simulink model "motor"  (R2017b)
settings: Solver=VariableStepAuto  StartTime=0.0  StopTime=10.0  RelTol=1e-3
values from neighbouring files (symbols this model uses):
  k1 = minium_chro(1)    [GA_fuzzy.m]    (also in GA_fuzzy_fitfun.m = chro(1))
  k2 = minium_chro(2)    [GA_fuzzy.m]    (also in GA_fuzzy_fitfun.m = chro(2))
libraries: fuzblock x1
settings Model: Creator=liyenjun  LastModifiedBy=liyenjun

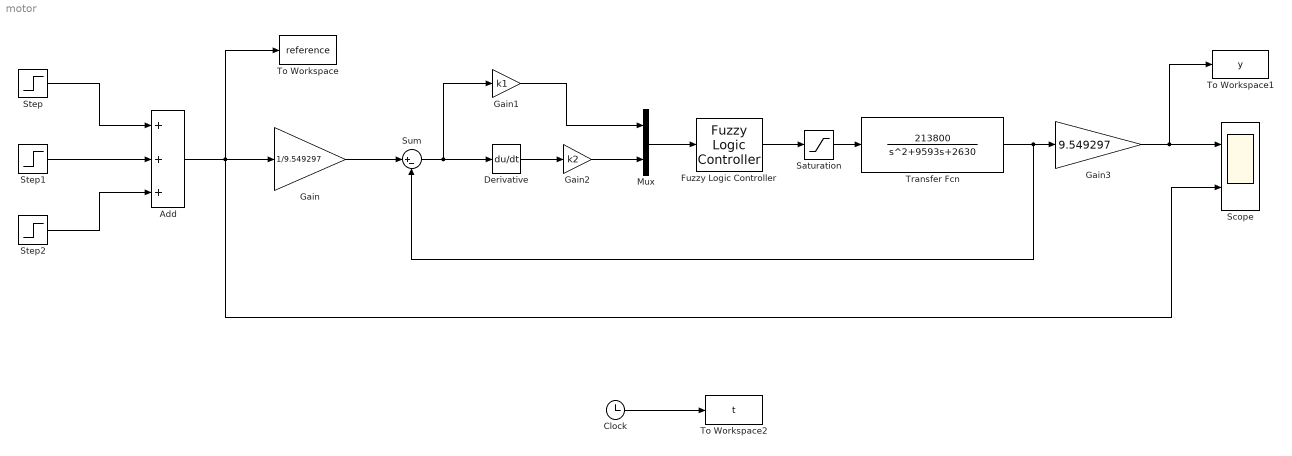
== system motor ==
  Add : Sum  Inputs=+++
  Clock : Clock
  Derivative : Derivative
  Fuzzy Logic Controller : fuzblock/Fuzzy Logic  Controller  FIS='tipper.fis'  OutputSampleNumber=101  DataType=double  FuzzifiedInputs=off  RuleFiringStrengths=off  RuleOutputs=off  AggregatedOutputs=off  SimulateUsing=Interpreted execution
  Gain : Gain  Gain=1/9.549297
  Gain1 : Gain  Gain=k1
  Gain2 : Gain  Gain=k2
  Gain3 : Gain  Gain=9.549297
  Mux : Mux  Inputs=2
  Saturation : Saturate
  Scope : Scope  NumInputPorts=2
  Step : Step  Before=1  SampleTime=0
  Step1 : Step  SampleTime=0
  Step2 : Step  Before=1  After=0  SampleTime=0
  Sum : Sum  Inputs=|+-
  To Workspace : ToWorkspace  VariableName=reference  SaveFormat=Timeseries  SampleTime=-1
  To Workspace1 : ToWorkspace  VariableName=y  SaveFormat=Timeseries  SampleTime=-1
  To Workspace2 : ToWorkspace  VariableName=t  SaveFormat=Timeseries  SampleTime=-1
  Transfer Fcn : TransferFcn  Numerator=[213800]  Denominator=[1 9593 2630]
  wires:
  Step/1 -> Add/1
  Step1/1 -> Add/2
  Step2/1 -> Add/3
  Add/1 -> To Workspace/1, Scope/2, Gain/1
  Gain/1 -> Sum/1
  Sum/1 -> Derivative/1, Gain1/1
  Derivative/1 -> Gain2/1
  Gain1/1 -> Mux/1
  Mux/1 -> Fuzzy Logic Controller/1
  Fuzzy Logic Controller/1 -> Saturation/1
  Saturation/1 -> Transfer Fcn/1
  Clock/1 -> To Workspace2/1
  Gain3/1 -> To Workspace1/1, Scope/1
  Transfer Fcn/1 -> Gain3/1, Sum/2
  Gain2/1 -> Mux/2
